simulink model "VelocityProfileStraightPath"  (R2023b)
settings: Solver=VariableStepAuto  StartTime=0.0  StopTime=10.0  RelTol=1e-3
values from neighbouring files (symbols this model uses):
  fwdorbwd = ones(arraylength,1)    [Parametersettingscript.m]    (also in Velocityprofiler_test.m)
  lengths = Routesegment(:,3)    [Parametersettingscript.m]    (also in Velocityprofiler_test.m)
  roadcurvatures = zeros(arraylength,1)    [Parametersettingscript.m]    (also in Velocityprofiler_test.m)
  V_end = 6    [Parametersettingscript.m]    (also in Velocityprofiler_test.m = 1)
  V_start = 0    [Parametersettingscript.m]    (also in Velocityprofiler_test.m = 30)
libraries: drivinglib x1
settings Model: Creator=The MathWorks, Inc.  LastModifiedBy=Jords
settings SolverCC: AlgebraicLoopSolver=TrustRegion
settings DataIOCC: SaveFormat=Structure
settings DebuggingCC: UnconnectedInputMsg=warning  UnconnectedOutputMsg=warning  UnconnectedLineMsg=warning  SymbolicDimsDataTypeCodeGenerationDiagnostic=none
settings ModelReferenceCC: EnableRefExpFcnMdlSchedulingChecks=on
settings SFSimCC: CustomCodeUndefinedFunction=UseInterfaceOnly
settings RTWCC: DLArmComputeVersion=19.05

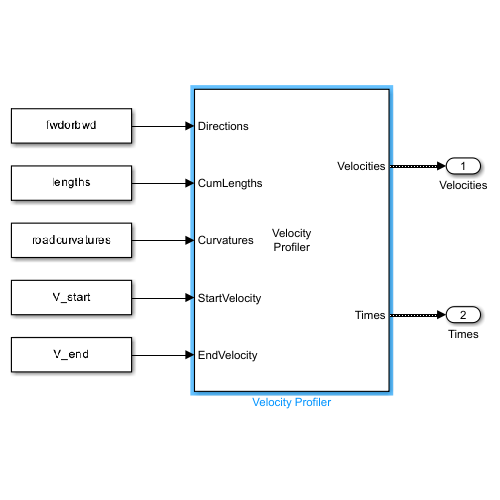
[thumbnail: Simulink's stored preview of the top-level diagram]
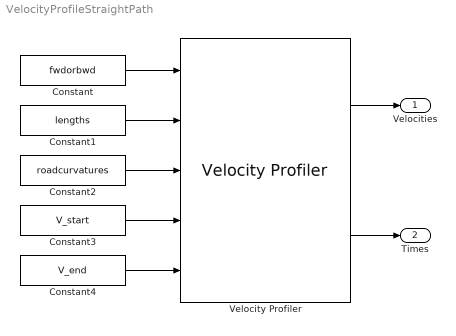
== system VelocityProfileStraightPath ==
  Constant : Constant  Value=fwdorbwd
  Constant1 : Constant  Value=lengths
  Constant2 : Constant  Value=roadcurvatures
  Constant3 : Constant  Value=V_start
  Constant4 : Constant  Value=V_end
  Velocity Profiler : drivinglib/Velocity Profiler  MaxLongitudinalAccel=maxlonacc  MaxLongitudinalDecel=maxlondec  MaxSpeed=maxspeed  MaxLongitudinalJerk=maxlonjerk  MaxLateralAccel=maxlatacc  ShowOptionalOutport=on  SampleTime=0.1  SimulateUsing=Code generation
  Velocities : Outport  VectorParamsAs1DForOutWhenUnconnected=off
  Times : Outport  Port=2  VectorParamsAs1DForOutWhenUnconnected=off
  wires:
  Constant/1 -> Velocity Profiler/1
  Constant1/1 -> Velocity Profiler/2
  Constant2/1 -> Velocity Profiler/3
  Constant3/1 -> Velocity Profiler/4
  Constant4/1 -> Velocity Profiler/5
  Velocity Profiler/1 -> Velocities/1
  Velocity Profiler/2 -> Times/1
